simulink model "EVnewtest"  (R2022b)
settings: Solver=VariableStepAuto  StartTime=0.0  StopTime=60  RelTol=1e-3
undefined symbols (not defined in the file): Ion, Lithium, sigbuilder_block
libraries: fl_lib x5, sdl_lib x5, nesl_utility x5, ee_lib x3, autolibshared x2, spsBatteryLib x1, spsControlledCurrentSourceLib x1, spspowerguiLib x1
(part 3 of 3)

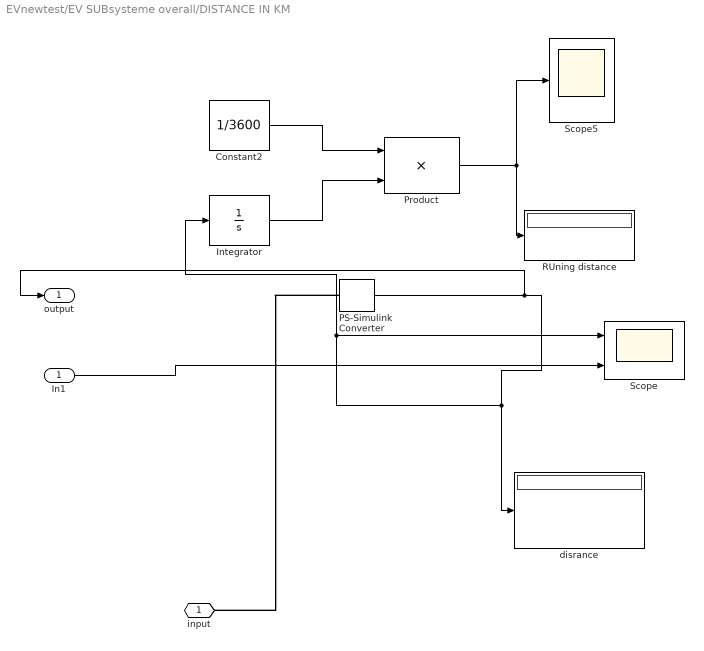
== system EVnewtest/EV SUBsysteme overall/DISTANCE IN KM ==
  In1 : Inport
  Constant2 : Constant  Value=1/3600
  Integrator : Integrator
  PS-Simulink Converter : nesl_utility/PS-Simulink Converter  PhysicalDomain=network_engine_domain  SubClassName=ps_output  LeftPortType=input  RightPortType=output  PseudoPeriodic=off  Frequencies=[]  VectorFormat=inherit  Unit=km/hr  AffineConversion=on
  Product : Product
  RUning distance : Display
  Scope : Scope  NumInputPorts=2
  Scope5 : Scope
  disrance : Display
  input : PMIOPort  Side=Left
  output : Outport
  wires:
  In1/1 -> Scope/2
  PS-Simulink Converter/1 -> output/1, disrance/1, Integrator/1, Scope/1
  Product/1 -> RUning distance/1, Scope5/1
  Constant2/1 -> Product/1
  Integrator/1 -> Product/2
  connections:
  PS-Simulink Converter/LConn1 -- input/RConn1

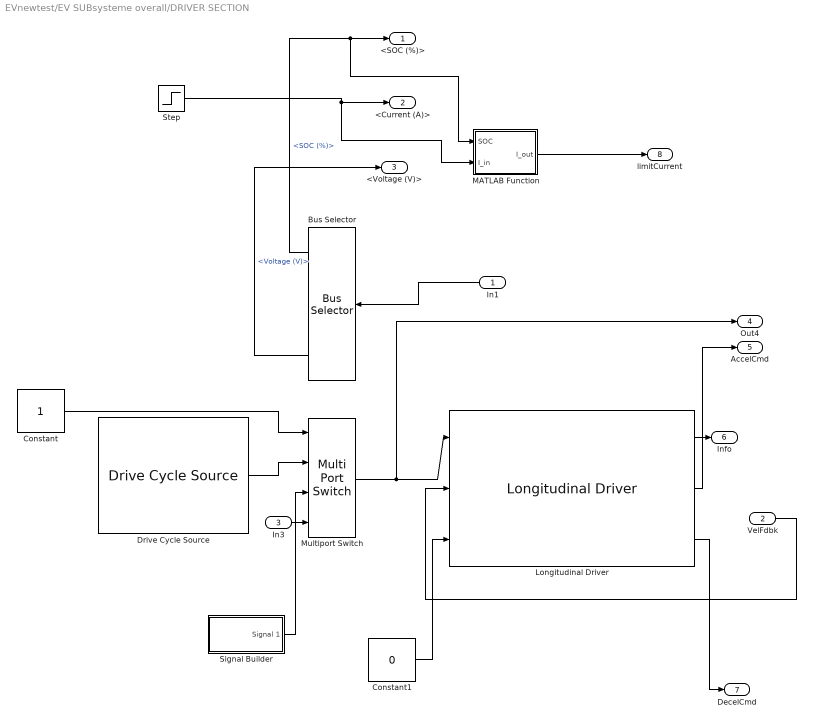
== system EVnewtest/EV SUBsysteme overall/DRIVER SECTION ==
  In1 : Inport
  VelFdbk : Inport  Port=2
  In3 : Inport  Port=3
  Bus Selector : BusSelector  OutputSignals=SOC (%),Current (A),Voltage (V)
  Constant : Constant
  Constant1 : Constant  Value=0
  Drive Cycle Source : autolibshared/Drive Cycle Source  cycleVar=.mat, .xls, .xlsx or .txt file  fileVar=cycleFTP75.mat  tfinal="2474  seconds"  cycleRepeat=off  outAccPort=off  outGearPort=off  gearList=No gear data  t_wot1=5  xdot_woto=0  xdot_wot1=30  t_wot2=20  xdot_wot2=0  t_wotend=30  srcUnit=m/s  outUnit=km/hr  srcAccUnit=m/s/s  outAccUnit=m/s^2  dt=0  aMode=1  faultOption=off  velBnd=2  velBndUnit=mph  inUnit=m/s  timeBnd=1  failOption=off  stopSim=off  maxFaultCnt=10  maxFaultTime=2  maxTotFaultTime=15  traceOption=off  dtTrace=1  traceWindow=10  lastDCname=Custom Data Set 1  lastOutUnit=mph  lastDT=0  lastTB=1  lastSB=2  forceCalcBound=off
  Longitudinal Driver : autolibshared/Longitudinal Driver  extAccelOvr=off  extDecelOvr=off  extAccelHld=off  extDecelHld=off  extAccelZero=off  extDecelZero=off  cntrlType=PI  shftType=None  velUnits=m/s  gearOut=off  Kp=10  Ki=5  Kff=.01  Kg=0  VehVelVec=[0 100]  KffVec=[.1 .1]  KpVec=[10 10]  KiVec=[5 5]  KgVec=[0 0]  m=1500  Kpt=3000  tau=.1  L=2  aR=200  bR=2.5  cR=.5  g=9.81  vnom=5  Kaw=1  tauerr=.01  tauPt=2  GearInit=0  tShift=.1  pdlVec=[0.1 0.4 0.5 0.9]  upShftTbl=[-1 12.9375 26.4375 39.9375 51.18749999999999 62.4375 72.84375 83.25;-1 16.3125 29.8125 43.3125 54.5624 65.8125 76.78125 87.75;-1 19.6875 33.1875 46.68749999999999 57.9375 69.1875 80.71875 92.25;-1 33 52.5 77.25 100.5 138.75 161.875 185]  dwnShftTbl=[1 9.5625 23.0625 36.5625 47.8125 59.0625 68.90625 78.75;1 12.9375 26.4375 39.9375 51.18749999999999 62.4375 72.84375 83.25;1 16.3125 29.8125 43.3125 54.562499 65.8125 76.78125 87.75;1 19.6875 33.1875 46.68749999999999 57.9375 69.1875 80.71875 92.25]  tClutch=.5  tRev=.5  tPark=120  aMode=2  UpGearVec="[0  1  2  3  4  5  6  7]"  DownGearVec="[1  2  3  4  5  6  7  8]"
      settings: LibrarySourceBlock=vehdynlibdriver/Longitudinal Driver
  MATLAB Function : MATLAB Function  TreatAsAtomicUnit=on
  Multiport Switch : MultiPortSwitch  SaturateOnIntegerOverflow=off  InputSameDT=off
  Signal Builder : Subsystem  Tag=STV Subsys  LoadFcn=sigbuilder_block('load');  StartFcn=sigbuilder_block('start');  StopFcn=sigbuilder_block('stop');  ClipboardFcn=sigbuilder_block('clipboard');  mask(Sigbuilder block){tuvar=[0:10]}
      mask help: Simulink:masks:SigbuilderBlock_MD
      mask init:
      | if ~strcmp(get_param(bdroot(gcbh),'SimulationStatus'),'stopped') tuvar = sigbuilder_block('maskInit'); end
      settings: CopyFcn=sigbuilder_block('copy');  DeleteFcn=sigbuilder_block('delete');  ModelCloseFcn=sigbuilder_block('modelClose');  PreSaveFcn=sigbuilder_block('preSave');  PauseFcn=sigbuilder_block('pause');  ContinueFcn=sigbuilder_block('continue');  NameChangeFcn=sigbuilder_block('namechange');  OpenFcn=sigbuilder_block('open',[437.6 199.2 550.4 400 ]);  CloseFcn=sigbuilder_block('close');
      mask Display: plot(0, 0, 100, 100,[2, 2, 32, 32, 2], [68, 8, 8, 68, 68],[32, 2], [38, 38], [32, 19, 2],[53, 60, 44], [32, 17, 17, 2],[16, 16, 31, 31]);txt = getActiveGroup(gcbh);text(2, 100, txt,'verticalAlignment', 'top');
  Step : Step  SampleTime=0
  <SOC (%)> : Outport
  <Current (A)> : Outport  Port=2
  <Voltage (V)> : Outport  Port=3
  Out4 : Outport  Port=4
  AccelCmd : Outport  Port=5
  Info : Outport  Port=6
  DecelCmd : Outport  Port=7
  limitCurrent : Outport  Port=8
  wires:
  Signal Builder/1(Signal 1) -> Multiport Switch/3
  Bus Selector/1 -> MATLAB Function/1(SOC), <SOC (%)>/1  "<SOC (%)>"
  Constant/1 -> Multiport Switch/1
  Longitudinal Driver/3 -> DecelCmd/1
  VelFdbk/1 -> Longitudinal Driver/2
  Constant1/1 -> Longitudinal Driver/3
  Longitudinal Driver/2 -> AccelCmd/1
  Multiport Switch/1 -> Out4/1, Longitudinal Driver/1
  Drive Cycle Source/1 -> Multiport Switch/2
  In1/1 -> Bus Selector/1
  Longitudinal Driver/1 -> Info/1
  Bus Selector/3 -> <Voltage (V)>/1  "<Voltage (V)>"
  Step/1 -> MATLAB Function/2(I_in), <Current (A)>/1
  In3/1 -> Multiport Switch/4
  MATLAB Function/1(I_out) -> limitCurrent/1

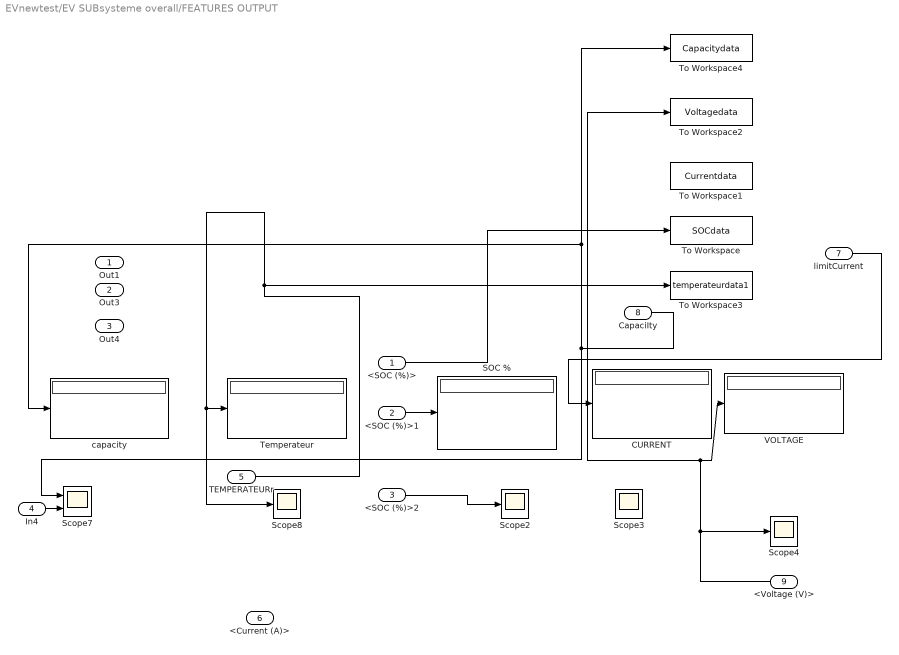
== system EVnewtest/EV SUBsysteme overall/FEATURES OUTPUT ==
  <SOC (%)> : Inport
  <SOC (%)>1 : Inport  Port=2
  <SOC (%)>2 : Inport  Port=3
  In4 : Inport  Port=4
  TEMPERATEURr : Inport  Port=5
  <Current (A)> : Inport  Port=6
  limitCurrent : Inport  Port=7
  CapaciIty : Inport  Port=8
  <Voltage (V)> : Inport  Port=9
  CURRENT : Display
  SOC % : Display
  Scope{2..4,8} (4 alike) : Scope
  Scope7 : Scope  NumInputPorts=2
  Temperateur : Display
  To Workspace : ToWorkspace  VariableName=SOCdata  SaveFormat=Timeseries  SampleTime=-1
  To Workspace1 : ToWorkspace  VariableName=Currentdata  SaveFormat=Timeseries  SampleTime=-1
  To Workspace2 : ToWorkspace  VariableName=Voltagedata  SaveFormat=Timeseries  SampleTime=-1
  To Workspace3 : ToWorkspace  VariableName=temperateurdata1  SaveFormat=Timeseries  SampleTime=-1
  To Workspace4 : ToWorkspace  VariableName=Capacitydata  SaveFormat=Timeseries  SampleTime=-1
  VOLTAGE : Display
  capacity : Display
  Out1 : Outport
  Out3 : Outport  Port=2
  Out4 : Outport  Port=3
  wires:
  CapaciIty/1 -> Scope7/1, To Workspace4/1, capacity/1
  <Voltage (V)>/1 -> VOLTAGE/1, To Workspace2/1, Scope4/1
  TEMPERATEURr/1 -> Scope8/1, Temperateur/1, To Workspace3/1
  <SOC (%)>2/1 -> Scope2/1
  In4/1 -> Scope7/2
  <SOC (%)>1/1 -> SOC %/1
  <SOC (%)>/1 -> To Workspace/1
  limitCurrent/1 -> CURRENT/1

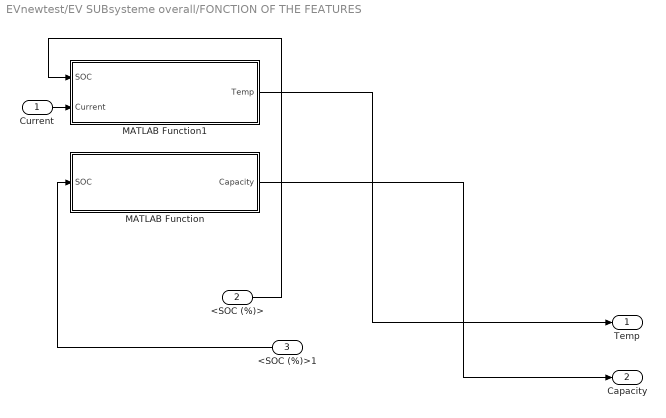
== system EVnewtest/EV SUBsysteme overall/FONCTION OF THE FEATURES ==
  Current : Inport
  <SOC (%)> : Inport  Port=2
  <SOC (%)>1 : Inport  Port=3
  MATLAB Function : MATLAB Function  TreatAsAtomicUnit=on
  MATLAB Function1 : MATLAB Function  TreatAsAtomicUnit=on
  Temp : Outport
  Capacity : Outport  Port=2
  wires:
  Current/1 -> MATLAB Function1/2(Current)
  <SOC (%)>/1 -> MATLAB Function1/1(SOC)
  MATLAB Function1/1(Temp) -> Temp/1
  MATLAB Function/1(Capacity) -> Capacity/1
  <SOC (%)>1/1 -> MATLAB Function/1(SOC)

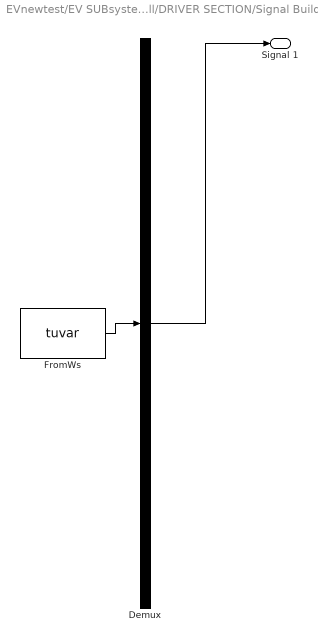
== system EVnewtest/EV SUBsysteme overall/DRIVER SECTION/Signal Builder ==
  Demux : Demux  Tag=STV Demux  Outputs=1
      settings: DisplayOption=none
  FromWs : FromWorkspace  Tag=STV FromWs  VariableName=tuvar
      SigBuilderData=|
      | common.afterFinalStr = 'Extrapolate'
      | common.sampleTime = 0
      | dataSet.timeRange = [0 10]
      | dataSet.name = 'Group 1'
      | sbobj.Groups.Name = 'Group 1'
      | sbobj.Groups.Signals.Name = 'Signal 1'
      | sbobj.Groups.Signals.XData = [0 4 4 6 6 10]
      | sbobj.Groups.Signals.YData = [0 0 1 1 0 0]
  Signal 1 : Outport  Tag=STV Outport
  wires:
  Demux/1 -> Signal 1/1
  FromWs/1 -> Demux/1

== matlab function EVnewtest/EV SUBsysteme overall/FONCTION OF THE FEATURES/MATLAB Function ==
  data: SOC input; Capacity output
function Capacity = getCapacity(SOC)
%#codegen

% This function converts State of Charge (%) to actual remaining Capacity (Ah)

% Define the nominal capacity of the battery (adjust as needed)
Nominal_Capacity = 100;  % [Ah] Example: 100Ah battery

% Convert SOC (%) to Capacity (Ah)
Capacity = (SOC / 100) * Nominal_Capacity;

end

== matlab function EVnewtest/EV SUBsysteme overall/DRIVER SECTION/MATLAB Function ==
  data: SOC input; I_out output; I_in input
function I_out = limitCurrent(SOC, I_in)
    rated_capacity = 50; % Ah
    max_c_rate = 2;      % e.g., 2C limit
    max_current = rated_capacity * max_c_rate; % = 100 A

    % Clamp the current value
    I_out = max(min(I_in, max_current), -max_current);
end

== matlab function EVnewtest/EV SUBsysteme overall/FONCTION OF THE FEATURES/MATLAB Function1 ==
  data: SOC input; Temp output; Current input
function Temp = estimateTemperature(SOC, Current)
% Simulated thermal model using SOC and current load

T_min = 25;
T_max = 60;

% Heating factor based on discharge
load_heat = abs(Current) * 0.05;

% Temperature profile affected by SOC
Temp = T_max - (SOC / 100) * (T_max - T_min) + load_heat;
